simulink model "asynchr"  (R2013a)
settings: Solver=ode23tb  StartTime=0.0  StopTime=100  RelTol=1e-3
libraries: powerlib x4
settings Model: Creator=imane  LastModifiedBy=imane

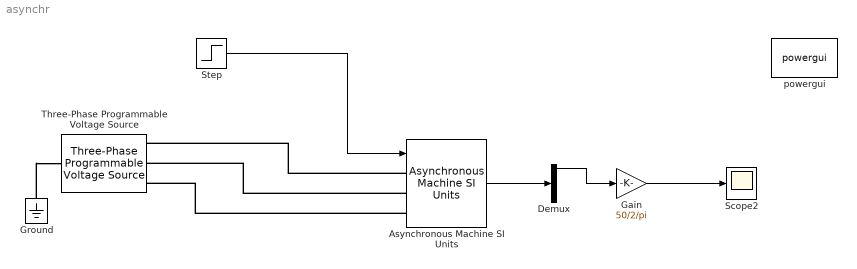
== system asynchr ==
  Asynchronous Machine SI Units : powerlib/Machines/Asynchronous Machine SI Units  PresetModel="17:  20 HP (15KW)   400 V 50Hz 1460 RPM"  MechanicalLoad=Torque Tm  ShowDetailedParameters=on  RotorType=Squirrel-cage  ReferenceFrame=Stationary  NominalParameters=[ 2250*746, 2400, 60 ]  Stator=[ 0.029 0.226/377]  Rotor=[ 0.022 0.226/377]  Cage1=[ 0.022 0.226/377]  Cage2=[ 0.022 0.226/377]  Lm=13.04/377  Mechanical="[ 63.87 0  2 ]"  PolePairs=2  InitialConditions=[1 0 0 0 0 0 0 0]  Units=SI  LoadFlowParameters=1492000  SimulateSaturation=off  Saturation=[14.03593122, 27.81365428, 53.79336849, 72.68890987, 97.98006896, 148.6815601, 215.7428561, 302.9841135, 420.4778367 ; 230, 322, 414, 460, 506, 552, 598, 644, 690]  TsPowergui=0  TsBlock=-1  IterativeModel=Trapezoidal non iterative  Pmec=0
  Demux : Demux
  Gain : Gain  Gain=50/2/pi
  Ground : powerlib/Elements/Ground  LConnTagsString=a
  Scope2 : Scope
  Step : Step  After=50  SampleTime=0
  Three-Phase Programmable Voltage Source : powerlib/Electrical Sources/Three-Phase Programmable Voltage Source  PositiveSequence="[400  0 50]"  VariationEntity=None  VariationType=Table of time-amplitude pairs  VariationTypeAlt=Step  VariationStep=0.5  VariationRate=10  VariationMagnitude=0.3  VariationFrequency=2  VariationTiming=[1 2]  VariationPhaseA=off  Amplitudes=[1 0.8 1.2 1.0]  TimeValues=[0 0.1 0.15 0.2]  HarmonicGeneration=off  HarmonicA=[3 0.2 -25 0]  HarmonicB=[2 0.15 35 2]  Timing="[0.05  3]"  BusType=swing  Pref=0  Qref=0  Qmin=-inf  Qmax=inf
  powergui : powerlib/powergui  Priority=1  SimulationMode=Continuous  SolverType=Tustin  SampleTime=50e-6  frequency=60  SPID=off  DisableSnubberDevices=off  DisableRonSwitches=off  DisableVfSwitches=off  SwTol=0  Interpol=off  DisplayEquations=off  frequencyindice=60  Pbase=100e6  ErrMax=1e-4  Iterations=50  UnitsV=kV  UnitsW=MW  FunctionMessages=off  echomessages=off  HookPort=off  EnableUseOfTLC=off  x0status=blocks  RestoreLinks=warning  ResistiveCurrentMeasurement=off  Frange=[0:2:500]  Ylog=off  Xlog=on  ShowGrid=off  save=off  variable=ZData  ZoomFFT=off  StartTime=0.0  cycles=1  DisplayStyle=1  fundamental=60  FreqAxis=off  MaxFrequency=1000  frequencyindicesteady=1  RmsSteady=1  display=off  Ts=0  methode=off
  wires:
  Step/1 -> Asynchronous Machine SI Units/1
  Gain/1 -> Scope2/1
  Asynchronous Machine SI Units/1 -> Demux/1
  Demux/1 -> Gain/1
  connections:
  Asynchronous Machine SI Units/LConn2 -- Three-Phase Programmable Voltage Source/RConn2
  Asynchronous Machine SI Units/LConn3 -- Three-Phase Programmable Voltage Source/RConn3
  Asynchronous Machine SI Units/LConn1 -- Three-Phase Programmable Voltage Source/RConn1
  Ground/LConn1 -- Three-Phase Programmable Voltage Source/LConn1
